simulink subsystem "MPC1_nlpsol_qrqp"  (R2023b)
settings: Solver=VariableStepAuto  StartTime=0.0  StopTime=10.0  RelTol=1e-3
undefined symbols (not defined in the file): param_MPC1, param_MPC1_traj_data, param_weight_MPC1
settings Model: Creator=emu  LastModifiedBy=emu

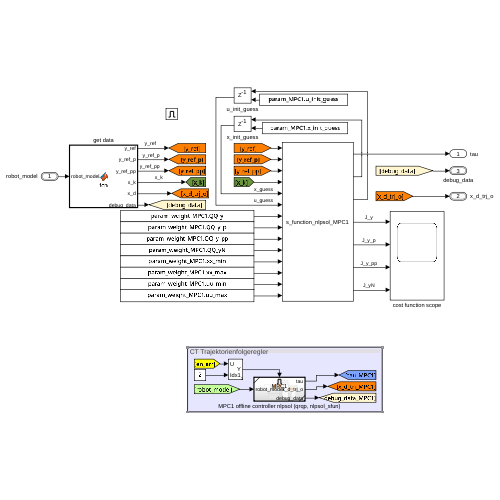
[thumbnail: Simulink's stored preview of the top-level diagram]
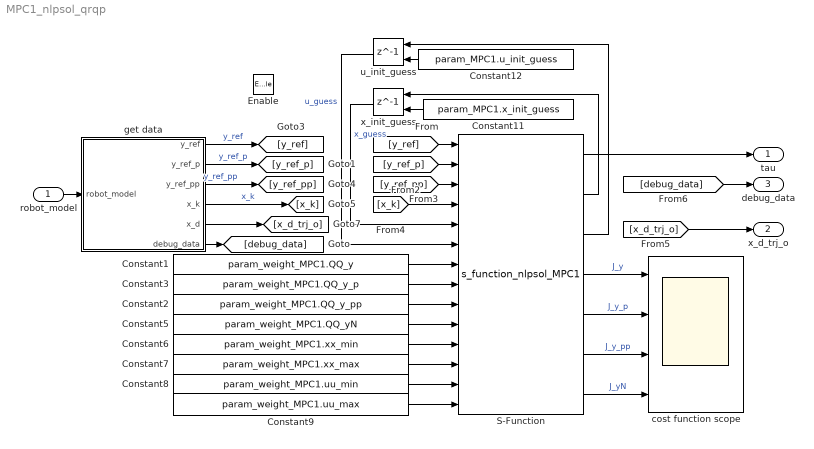
== system MPC1_nlpsol_qrqp ==
  robot_model : Inport  OutDataTypeStr=Bus: robot_model
  Enable : EnablePort
  Constant1 : Constant  Value=param_weight_MPC1.QQ_y
  Constant11 : Constant  Value=param_MPC1.x_init_guess
  Constant12 : Constant  Value=param_MPC1.u_init_guess
  Constant2 : Constant  Value=param_weight_MPC1.QQ_y_pp
  Constant3 : Constant  Value=param_weight_MPC1.QQ_y_p
  Constant5 : Constant  Value=param_weight_MPC1.QQ_yN
  Constant6 : Constant  Value=param_weight_MPC1.xx_min
  Constant7 : Constant  Value=param_weight_MPC1.xx_max
  Constant8 : Constant  Value=param_weight_MPC1.uu_min
  Constant9 : Constant  Value=param_weight_MPC1.uu_max
  S-Function : S-Function  FunctionName=s_function_nlpsol_MPC1  Parameters='s_functions/MPC1.casadi', 'MPC1'  SFunctionDeploymentMode=off  EnableBusSupport=off
  cost function scope : Scope  NumInputPorts=4
  get data : MATLAB Function  TreatAsAtomicUnit=on
  u_init_guess : Delay  DelayLength=1  InitialConditionSource=Input port  InitialCondition=1
      settings: InputPortMap=u0,p4
  x_init_guess : Delay  DelayLength=1  InitialConditionSource=Input port  InitialCondition=1
      settings: InputPortMap=u0,p4
  tau : Outport
  x_d_trj_o : Outport  Port=2  OutDataTypeStr=Bus: x_d
  debug_data : Outport  Port=3  OutDataTypeStr=Bus: debug_data_bus
  wires:
  S-Function/4 -> cost function scope/1  "J_y"
  [debug_data] -> debug_data/1
  [y_ref_p] -> S-Function/2
  Constant7/1 -> S-Function/12
  Constant9/1 -> S-Function/14
  [y_ref_pp] -> S-Function/3
  [x_d_trj_o] -> x_d_trj_o/1
  S-Function/3 -> u_init_guess/1
  get data/4(x_k) -> [x_k]  "x_k"
  get data/3(y_ref_pp) -> [y_ref_pp]  "y_ref_pp"
  Constant12/1 -> u_init_guess/2
  get data/2(y_ref_p) -> [y_ref_p]  "y_ref_p"
  get data/1(y_ref) -> [y_ref]  "y_ref"
  Constant11/1 -> x_init_guess/2
  [y_ref] -> S-Function/1
  [x_k] -> S-Function/4
  S-Function/2 -> x_init_guess/1
  x_init_guess/1 -> S-Function/5  "x_guess"
  get data/6(debug_data) -> [debug_data]
  u_init_guess/1 -> S-Function/6  "u_guess"
  get data/5(x_d) -> [x_d_trj_o]
  S-Function/7 -> cost function scope/4  "J_yN"
  S-Function/6 -> cost function scope/3  "J_y_pp"
  Constant2/1 -> S-Function/9
  Constant5/1 -> S-Function/10
  Constant3/1 -> S-Function/8
  S-Function/5 -> cost function scope/2  "J_y_p"
  robot_model/1 -> get data/1(robot_model)
  S-Function/1 -> tau/1
  Constant1/1 -> S-Function/7
  Constant6/1 -> S-Function/11
  Constant8/1 -> S-Function/13

== matlab function MPC1_nlpsol_qrqp/get data ==
  settings: updateMethod=DISCRETE  sampleTime=param_global.Ta
  data: y_ref output; robot_model input Bus: robot_model; param_MPC1 parameter; y_ref_p output; y_ref_pp output; x_k output; x_d output Bus: x_d; debug_data output Bus: debug_data_bus; param_MPC1_traj_data parameter
function [y_ref, y_ref_p, y_ref_pp, x_k, x_d, debug_data] = fcn(robot_model, param_MPC1, param_MPC1_traj_data)
persistent cnt;

if(isempty(cnt))
    cnt = 1;
end

param_trajectory = param_MPC1_traj_data;
param_MPC = param_MPC1;
N         = param_MPC.N;
N_step    = param_MPC.N_step;

% Parameters
q    = robot_model.q;      % generalized coordinates
q_p  = robot_model.q_p;  % time derivative of generalized coordinates
q_pp = robot_model.q_pp;
H    = robot_model.H;
J    = robot_model.J;
J_p  = robot_model.J_p;

% Current Pose of Endeffector
p = H(1:2,4);
p_p = J(1:2,1:2)*q_p;
p_pp = J(1:2,1:2)*q_pp + J_p(1:2,1:2)*q_p;

R = H(1:3,1:3);

% desired Orientation as Rotationmatrix
q_e = rotation2quaternion(R);

% Error of Position (translation) and first time derivative
q_err = quat_mult(q_e, quat_inv(param_trajectory.q_d(:, cnt)));

x_k = [q;q_p];

% Assemble vector of recieved output measurements
p_d_traj    = param_trajectory.p_d(   1:3, cnt : N_step : cnt + N*(N_step  ));
p_d_p_traj  = param_trajectory.p_d_p( 1:3, cnt : N_step : cnt + N*(N_step-1));
p_d_pp_traj = param_trajectory.p_d_pp(1:3, cnt : N_step : cnt + N*(N_step-1));

y_ref    = p_d_traj(   1:2, 2:N+1); %y1, y2, ... yN
y_ref_p  = p_d_p_traj( 1:2, 2:N);   %y1_p, y2p, ... yN-1p
y_ref_pp = p_d_pp_traj(1:2, 2:N);   %y1_pp, y2pp, ... yN-1pp

cnt = cnt+1;

%% TRAJECTORY OUT
x_d.p_d       = p_d_traj(1:3,1);    %y0
x_d.p_d_p     = p_d_p_traj(1:3,1);  %y0p
x_d.p_d_pp    = p_d_pp_traj(1:3,1); %y0pp
x_d.q_d       = [0; 0; 0; 0];
x_d.omega_d   = [0; 0; 0];
x_d.omega_d_p = [0; 0; 0];

%% DEBUG
debug_data.p    = p(1:2);
debug_data.p_p  = p_p(1:2);
debug_data.p_pp = p_pp(1:2);
debug_data.rot_x_err = q_err(2);
debug_data.rot_y_err = q_err(3);
debug_data.rot_z_err = q_err(4);
